simulink model "l6p2"  (R2022a)
settings: Solver=VariableStepAuto  StartTime=0.0  StopTime=Tmdl  FixedStep=Ts  MaxStep=Ts  RelTol=1e-3
undefined symbols (not defined in the file or in its folder): im_m, kps
libraries: fl_lib x10, nesl_utility x7
settings Model: Creator=hdu  LastModifiedBy=86156

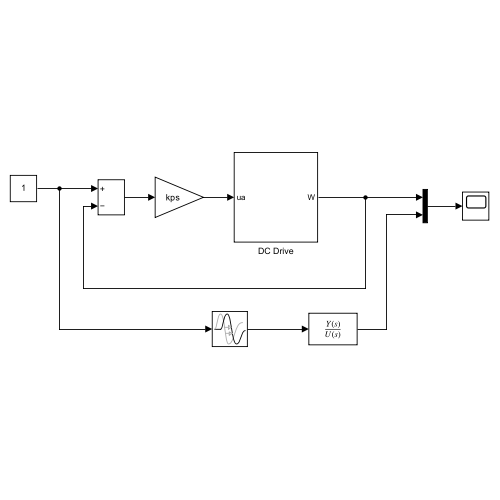
[thumbnail: Simulink's stored preview of the top-level diagram]
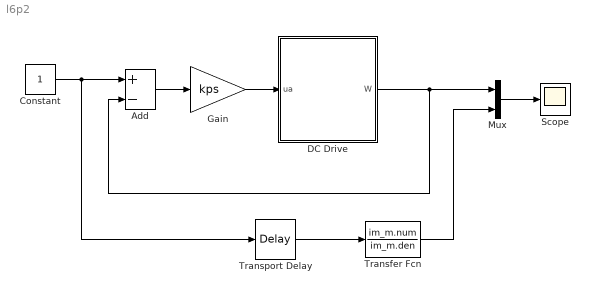
== system l6p2 ==
  Add : Sum  Inputs=+-
  Constant : Constant
  DC Drive : Subsystem
  Gain : Gain  Gain=kps
  Mux : Mux  Inputs=2
  Scope : Scope
  Transfer Fcn : TransferFcn  Numerator=im_m.num  Denominator=im_m.den
  Transport Delay : TransportDelay  DelayTime=0.001
  wires:
  Constant/1 -> Transport Delay/1, Add/1
  Transport Delay/1 -> Transfer Fcn/1
  DC Drive/1(W) -> Add/2, Mux/1
  Mux/1 -> Scope/1
  Transfer Fcn/1 -> Mux/2
  Add/1 -> Gain/1
  Gain/1 -> DC Drive/1(ua)

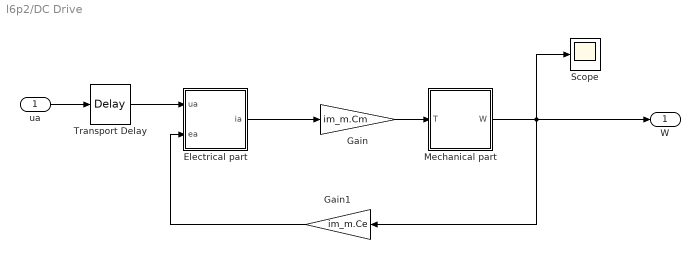
== system l6p2/DC Drive ==
  ua : Inport
  Electrical part : Subsystem
  Gain : Gain  Gain=im_m.Cm
  Gain1 : Gain  Gain=im_m.Ce
  Mechanical part : Subsystem
  Scope : Scope
  Transport Delay : TransportDelay  DelayTime=0.001
  W : Outport
  wires:
  Electrical part/1(ia) -> Gain/1
  Gain/1 -> Mechanical part/1(T)
  Transport Delay/1 -> Electrical part/1(ua)
  Gain1/1 -> Electrical part/2(ea)
  Mechanical part/1(W) -> W/1, Scope/1, Gain1/1
  ua/1 -> Transport Delay/1

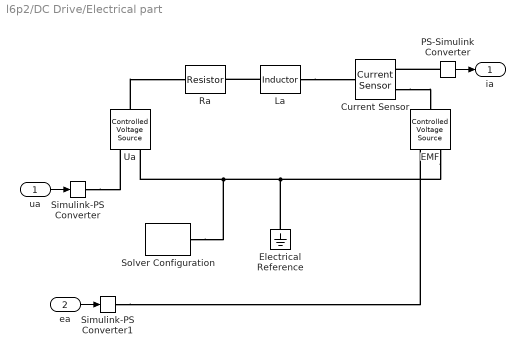
== system l6p2/DC Drive/Electrical part ==
  ua : Inport
  ea : Inport  Port=2
  Current Sensor : fl_lib/Electrical/Electrical Sensors/Current Sensor
  EMF : fl_lib/Electrical/Electrical Sources/Controlled Voltage Source
  Electrical Reference : fl_lib/Electrical/Electrical Elements/Electrical Reference
  La : fl_lib/Electrical/Electrical Elements/Inductor  l=im_m.L H  r=0 Ohm  g=1e-9 1/Ohm  i_specify=off  i_priority=None  i=0 A  i_nominal_specify=off  i_nominal_unit=A  i_nominal_value=1  v_specify=off  v_priority=None  v=0 V  v_nominal_specify=off  v_nominal_unit=V  v_nominal_value=1  i_L_specify=off  i_L_priority=High  i_L=0 A  i_L_nominal_specify=off  i_L_nominal_unit=A  i_L_nominal_value=1
  PS-Simulink Converter : nesl_utility/PS-Simulink Converter  PhysicalDomain=network_engine_domain  SubClassName=ps_output  LeftPortType=input  RightPortType=output  PseudoPeriodic=off  Frequencies=[]  VectorFormat=1-D array  Unit=inherit  AffineConversion=off
  Ra : fl_lib/Electrical/Electrical Elements/Resistor  R=im_m.R Ohm  i_specify=off  i_priority=None  i=0 A  i_nominal_specify=off  i_nominal_unit=A  i_nominal_value=1  v_specify=off  v_priority=None  v=0 V  v_nominal_specify=off  v_nominal_unit=V  v_nominal_value=1
  Simulink-PS Converter : nesl_utility/Simulink-PS Converter  PhysicalDomain=network_engine_domain  SubClassName=ps_input  LeftPortType=input  RightPortType=output  PseudoPeriodic=off  Frequencies=[]  NoiseDistribution=none  NoiseParameters=[]  Unit=1  AffineConversion=off  FilteringAndDerivatives=provide  SimscapeFilterOrder=1  InputFilterTimeConstant=0.001  UdotUserProvided=0
  Simulink-PS Converter1 : nesl_utility/Simulink-PS Converter  PhysicalDomain=network_engine_domain  SubClassName=ps_input  LeftPortType=input  RightPortType=output  PseudoPeriodic=off  Frequencies=[]  NoiseDistribution=none  NoiseParameters=[]  Unit=1  AffineConversion=off  FilteringAndDerivatives=provide  SimscapeFilterOrder=1  InputFilterTimeConstant=0.001  UdotUserProvided=0
  Solver Configuration : nesl_utility/Solver Configuration  PhysicalDomain=network_engine_domain  SubClassName=solver  LeftPortType=input  RightPortType=generic  Tones=[]  Harmonics=[]  SimulateNoise=off  Profile=off  UseLocalSampling=off  EnableSwitchedLinearOptims=on  FrequencyDomain=off  UseCCode=off  RelTol=0.001  AbsTol=1e-06  MinStep=1e-09  ToWorkspace=off  RevertToSquareIcSolve=off  NumHomotopyIterations=100  PhasorMode=off  PhasorModeNumHarmonics=1  ConsistencySolver=NEWTON_FTOL  IndexReductionMethod=DerivativeReplacement  DoDC=off  ResidualTolerance=1e-09  ConsistencyTolSource=GLOBAL  ConsistencyAbsTol=0.001  ConsistencyRelTol=0.001  ConsistencyTolFactor=0.001  UseLocalSolver=off  LocalSolverChoice=NE_BACKWARD_EULER_ADVANCER  ResolveIndetEquations=on  FunctionEvalNumThread=1  LocalSolverSampleTime=0.001  DoFixedCost=off  MaxNonlinIter=3  MaxModeIter=2  ComputeImpulses=off  ImpulseIterations=2  LinearAlgebra=auto  LinearAlgebraNumThread=0  EquationFormulation=NE_TIME_EF  DelaysMemoryBudget=1024  AutomaticFiltering=on  FilteringTimeConstant=0.001  PartitionStorageMethod=AS_NEEDED  PartitionMemoryBudget=1024  PartitionMethod=ROBUST
  Ua : fl_lib/Electrical/Electrical Sources/Controlled Voltage Source
  ia : Outport
  wires:
  ua/1 -> Simulink-PS Converter/1
  PS-Simulink Converter/1 -> ia/1
  ea/1 -> Simulink-PS Converter1/1
  connections:
  EMF/RConn2 -- Electrical Reference/LConn1 -- Solver Configuration/RConn1 -- Ua/RConn2
  Simulink-PS Converter/RConn1 -- Ua/RConn1
  Simulink-PS Converter1/RConn1 -- EMF/RConn1
  Current Sensor/RConn2 -- EMF/LConn1
  Ua/LConn1 -- Ra/LConn1
  La/LConn1 -- Ra/RConn1
  La/RConn1 -- Current Sensor/LConn1
  PS-Simulink Converter/LConn1 -- Current Sensor/RConn1

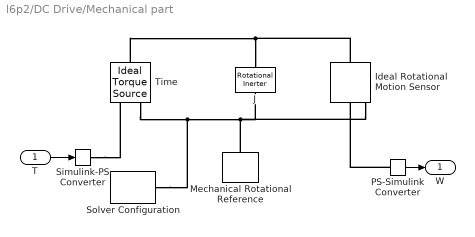
== system l6p2/DC Drive/Mechanical part ==
  T : Inport
  Ideal Rotational Motion Sensor : fl_lib/Mechanical/Mechanical Sensors/Ideal Rotational Motion Sensor  reference=foundation.enum.MeasurementReference.difference  acceleration_port=false  velocity_port=true  position_port=true  wrap_angle=simscape.enum.onoff.off  offset=0 rad
  J : fl_lib/Mechanical/Rotational Elements/Rotational Inerter  B=im_m.J kg*m^2  w_specify=off  w_priority=High  w=0 rad/s  w_nominal_specify=off  w_nominal_unit=rad/s  w_nominal_value=1  t_specify=off  t_priority=None  t=0 N*m  t_nominal_specify=off  t_nominal_unit=N*m  t_nominal_value=1
      settings: InternalSimscapePortConfiguration="{\"Bottom\":[],\"Left\":[{\"id\":\"R\",\"label\":\"R\",\"type\":\"foundation.mechanical.rotational.rotational\"}],\"Right\":[{\"id\":\"C\",\"label\":\"C\",\"type\":\"foundation.mechanical.rotational.rotational\"}],\"Top\":[]}"
  Mechanical Rotational Reference : fl_lib/Mechanical/Rotational Elements/Mechanical Rotational Reference
  PS-Simulink Converter : nesl_utility/PS-Simulink Converter  PhysicalDomain=network_engine_domain  SubClassName=ps_output  LeftPortType=input  RightPortType=output  PseudoPeriodic=off  Frequencies=[]  VectorFormat=1-D array  Unit=inherit  AffineConversion=off
  Simulink-PS Converter : nesl_utility/Simulink-PS Converter  PhysicalDomain=network_engine_domain  SubClassName=ps_input  LeftPortType=input  RightPortType=output  PseudoPeriodic=off  Frequencies=[]  NoiseDistribution=none  NoiseParameters=[]  Unit=1  AffineConversion=off  FilteringAndDerivatives=provide  SimscapeFilterOrder=1  InputFilterTimeConstant=0.001  UdotUserProvided=0
  Solver Configuration : nesl_utility/Solver Configuration  PhysicalDomain=network_engine_domain  SubClassName=solver  LeftPortType=input  RightPortType=generic  Tones=[]  Harmonics=[]  SimulateNoise=off  Profile=off  UseLocalSampling=off  EnableSwitchedLinearOptims=on  FrequencyDomain=off  UseCCode=off  RelTol=0.001  AbsTol=1e-06  MinStep=1e-09  ToWorkspace=off  RevertToSquareIcSolve=off  NumHomotopyIterations=100  PhasorMode=off  PhasorModeNumHarmonics=1  ConsistencySolver=NEWTON_FTOL  IndexReductionMethod=DerivativeReplacement  DoDC=off  ResidualTolerance=1e-09  ConsistencyTolSource=GLOBAL  ConsistencyAbsTol=0.001  ConsistencyRelTol=0.001  ConsistencyTolFactor=0.001  UseLocalSolver=off  LocalSolverChoice=NE_BACKWARD_EULER_ADVANCER  ResolveIndetEquations=on  FunctionEvalNumThread=1  LocalSolverSampleTime=0.001  DoFixedCost=off  MaxNonlinIter=3  MaxModeIter=2  ComputeImpulses=off  ImpulseIterations=2  LinearAlgebra=auto  LinearAlgebraNumThread=0  EquationFormulation=NE_TIME_EF  DelaysMemoryBudget=1024  AutomaticFiltering=on  FilteringTimeConstant=0.001  PartitionStorageMethod=AS_NEEDED  PartitionMemoryBudget=1024  PartitionMethod=ROBUST
  Time : fl_lib/Mechanical/Mechanical Sources/Ideal Torque Source
  W : Outport
  wires:
  PS-Simulink Converter/1 -> W/1
  T/1 -> Simulink-PS Converter/1
  connections:
  Time/LConn1 -- Ideal Rotational Motion Sensor/LConn1 -- J/LConn1
  PS-Simulink Converter/LConn1 -- Ideal Rotational Motion Sensor/RConn2
  Time/RConn2 -- Solver Configuration/RConn1 -- Ideal Rotational Motion Sensor/RConn1 -- J/RConn1 -- Mechanical Rotational Reference/LConn1
  Simulink-PS Converter/RConn1 -- Time/RConn1
